simulink model "ConstantCalc"  (R2022b)
settings: Solver=VariableStepAuto  StartTime=0.0  StopTime=10.0  RelTol=1e-3
settings Model: Creator=tilog  LastModifiedBy=tilog

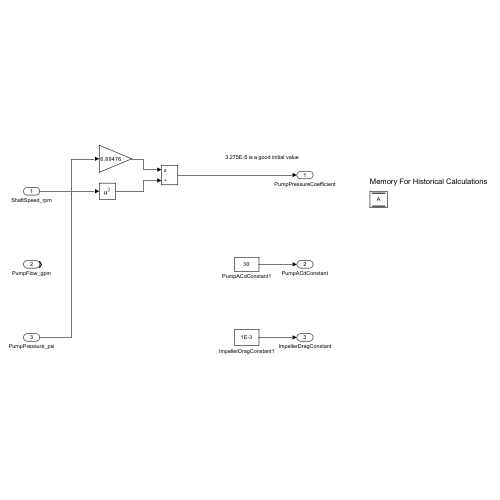
[thumbnail: Simulink's stored preview of the top-level diagram]
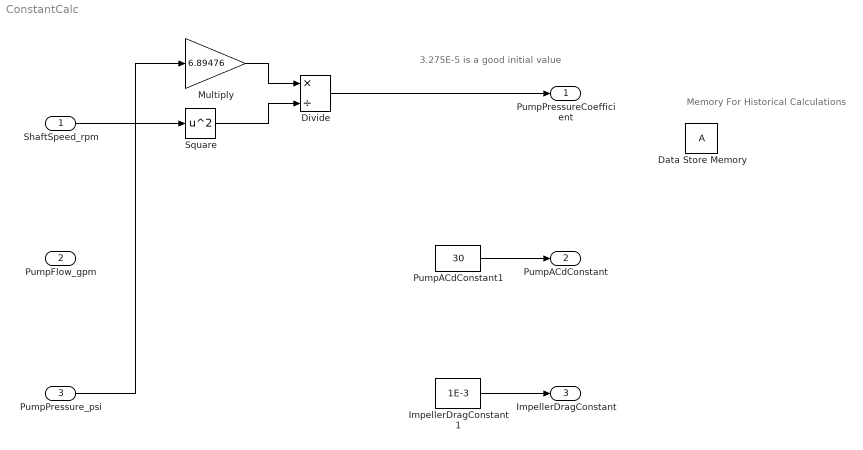
== system ConstantCalc ==
  note: Memory For Historical Calculations
  note: 3.275E-5 is a good initial value
  ShaftSpeed_rpm : Inport
  PumpFlow_gpm : Inport  Port=2
  PumpPressure_psi : Inport  Port=3
  Data Store Memory : DataStoreMemory  WriteAfterWriteMsg=warning  ShowAdditionalParam=off
  Divide : Product  Inputs=*/
  ImpellerDragConstant1 : Constant  Value=1E-3
  Multiply : Gain  Gain=6.89476
  PumpACdConstant1 : Constant  Value=30
  Square : Math  Operator=square
  PumpPressureCoefficient : Outport
  PumpACdConstant : Outport  Port=2
  ImpellerDragConstant : Outport  Port=3
  wires:
  ShaftSpeed_rpm/1 -> Square/1
  PumpPressure_psi/1 -> Multiply/1
  Square/1 -> Divide/2
  Multiply/1 -> Divide/1
  Divide/1 -> PumpPressureCoefficient/1
  ImpellerDragConstant1/1 -> ImpellerDragConstant/1
  PumpACdConstant1/1 -> PumpACdConstant/1
